simulink model "Cooperative"  (R2023b)
settings: Solver=FixedStepAuto  StartTime=0.0  StopTime=Sim_time  FixedStep=dt  RelTol=1e-3
values from neighbouring files (symbols this model uses):
  delta_r_max = 30*pi/180    (= 0.523598775598)    [Run_Cooperation.m]
  DS = 1    [Run_Cooperation.m]
  M_psi_r = 20*pi/180    (= 0.349065850399)    [Run_Cooperation.m]
  MaxF = 45    [Run_Cooperation.m]
  MinF = 15    [Run_Cooperation.m]
  SR = 30    [Run_Cooperation.m]
  targetX = [100,110,80,95]    [Run_Cooperation.m]
  targetY = [100, 120,130,125]    [Run_Cooperation.m]
  tau_s = 1    [Run_Cooperation.m]
  u0 = 1    [Run_Cooperation.m]
  xAUV_ini = [2, 15, 6, 20]    [Run_Cooperation.m]
  Xob = [35,50,80,50]    [Run_Cooperation.m]
  yAUV_ini = [15, -20, -5, 0]    [Run_Cooperation.m]
  Yob = [35,50,80,100]    [Run_Cooperation.m]
libraries: slpidlib x4, simulink x4
settings Model: Creator=Behnaz Hadi  LastModifiedBy=ps22aae
settings SolverCC: AlgebraicLoopSolver=TrustRegion
settings DataIOCC: ReturnWorkspaceOutputs=off
settings DebuggingCC: UnconnectedInputMsg=warning  UnconnectedOutputMsg=warning  UnconnectedLineMsg=warning  ArithmeticOperatorsInVariantConditions=warning
settings ModelReferenceCC: EnableRefExpFcnMdlSchedulingChecks=on
settings SFSimCC: CustomCodeUndefinedFunction=UseInterfaceOnly
settings RTWCC: DLArmComputeVersion=19.05

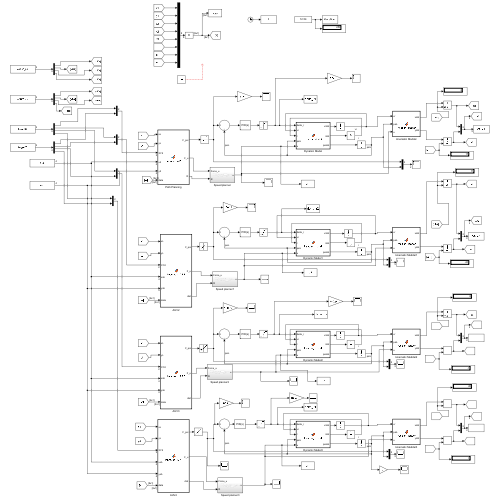
[thumbnail: Simulink's stored preview of the top-level diagram]
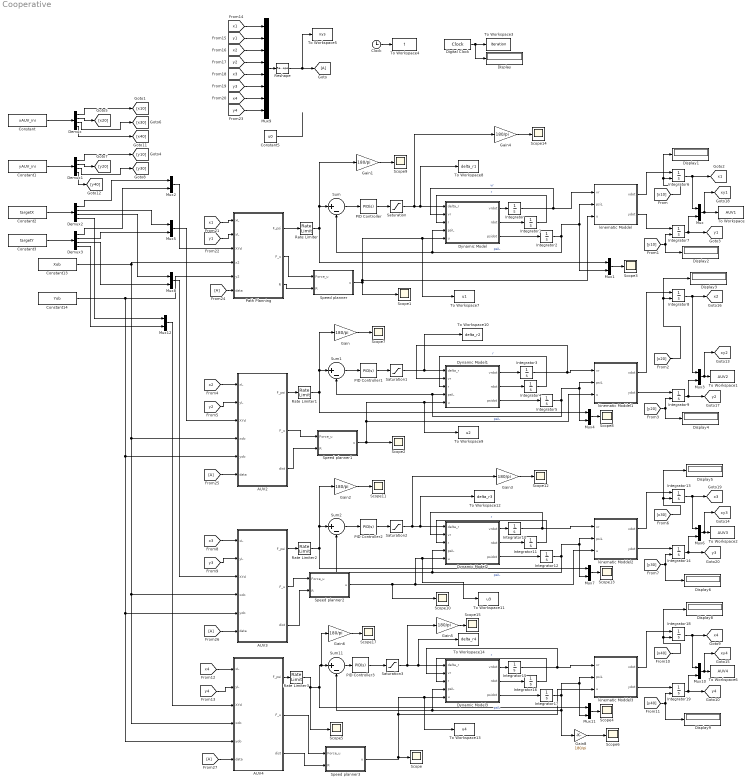
== system Cooperative ==
  AUV2 : MATLAB Function  TreatAsAtomicUnit=on
  AUV3 : MATLAB Function  TreatAsAtomicUnit=on
  AUV4 : MATLAB Function  TreatAsAtomicUnit=on
  Clock : Clock
  Constant : Constant  Value=xAUV_ini
  Constant1 : Constant  Value=yAUV_ini
  Constant13 : Constant  Value=Xob
  Constant14 : Constant  Value=Yob
  Constant2 : Constant  Value=targetX
  Constant3 : Constant  Value=targetY
  Constant5 : Constant  Value=u0
  Demux{,1..3} (4 alike) : Demux
  Digital Clock : DigitalClock
  Display{,1..6,8..9} (9 alike) : Display
  Dynamic Model : MATLAB Function  TreatAsAtomicUnit=on
  Dynamic Model1 : MATLAB Function  TreatAsAtomicUnit=on
  Dynamic Model2 : MATLAB Function  TreatAsAtomicUnit=on
  Dynamic Model3 : MATLAB Function  TreatAsAtomicUnit=on
  From{24..27} (4 alike) : From
  Gain{,1..6,8} (8 alike) : Gain  Gain=180/pi
  Goto : Goto
  Integrator{,1,3..4,10..11,15..16} (8 alike) : Integrator
  Integrator{2,5,12,17} (4 alike) : Integrator  InitialCondition=pi/6
  Integrator{6,8,13,18} (4 alike) : Integrator  InitialConditionSource=external  InitialCondition=6
  Integrator{7,9,14,19} (4 alike) : Integrator  InitialConditionSource=external  InitialCondition=4
  Mux{,1..8,10..12} (12 alike) : Mux  Inputs=2
  Mux9 : Mux  Inputs=8
  PID Controller{,1..3} (4 alike) : slpidlib/PID Controller  Controller=PID  Form=Ideal  TimeDomain=Continuous-time  UseExternalTs=off  SampleTime=-1  IntegratorMethod=Forward Euler  FilterMethod=Forward Euler  ControllerParametersSource=internal  P=-4.58375331776641  I=0.348826037798542  UseKiTs=off  D=0.667672634240164  N=10.0336095861132  UseFilter=on  TunerSelectOption=Transfer Function Based (PID Tuner App)  InitialConditionSource=internal  InitialConditionForIntegrator=0  InitialConditionForFilter=0  DifferentiatorICPrevScaledInput=0  ExternalReset=none  TrackingMode=off  Kt=1  LimitOutput=off  SatLimitsSource=internal  UpperSaturationLimit=inf  LowerSaturationLimit=-inf  LinearizeAsGain=on  AntiWindupMode=none  Kb=1  LimitIntegrator=off  UpperIntegratorSaturationLimit=inf  LowerIntegratorSaturationLimit=-inf  POutMin=[]  POutMax=[]  IOutMin=[]  IOutMax=[]  DOutMin=[]  DOutMax=[]  NOutMin=[]  NOutMax=[]  SumOutMin=[]  SumOutMax=[]  SaturationOutMin=[]  SaturationOutMax=[]  PParamMin=[]  PParamMax=[]  IParamMin=[]  IParamMax=[]  DParamMin=[]  DParamMax=[]  NParamMin=[]  NParamMax=[]  KbParamMin=[]  KbParamMax=[]  KtParamMin=[]  KtParamMax=[]  KbOutMin=[]  KbOutMax=[]  KtOutMin=[]  KtOutMax=[]  IntegratorOutMin=[]  IntegratorOutMax=[]  FilterOutMin=[]  FilterOutMax=[]  SumI1OutMin=[]  SumI1OutMax=[]  SumI2OutMin=[]  SumI2OutMax=[]  SumI3OutMin=[]  SumI3OutMax=[]  SumI4OutMin=[]  SumI4OutMax=[]  SumDOutMin=[]  SumDOutMax=[]  DifferentiatorOutMin=[]  DifferentiatorOutMax=[]  FilterDiffOutCoefMin=[]  FilterDiffOutCoefMax=[]  ReciprocalOutMin=[]  ReciprocalOutMax=[]  SumDenOutMin=[]  SumDenOutMax=[]  SumNumOutMin=[]  SumNumOutMax=[]  DivideOutMin=[]  DivideOutMax=[]  UdiffTsProdOutMin=[]  UdiffTsProdOutMax=[]  NTsProdOutMin=[]  NTsProdOutMax=[]  UintegralTsProdOutMin=[]  UintegralTsProdOutMax=[]  UngainTsProdOutMin=[]  UngainTsProdOutMax=[]  ClampingZeroOutDataTypeStr=Inherit: Inherit via back propagation  ClampingZeroOutMin=[]  ClampingZeroOutMax=[]  FilterDenConstantOutDataTypeStr=Inherit: Inherit via back propagation  FilterDenConstantOutMin=[]  FilterDenConstantOutMax=[]  PCopyOutDataTypeStr=Inherit: Inherit via back propagation  PCopyOutMin=[]  PCopyOutMax=[]  NCopyOutDataTypeStr=Inherit: Inherit via back propagation  NCopyOutMin=[]  NCopyOutMax=[]  IntegratorContinuousStateAttributes=''  IntegratorStateMustResolveToSignalObject=off  IntegratorRTWStateStorageClass=Auto  FilterContinuousStateAttributes=''  FilterStateMustResolveToSignalObject=off  FilterRTWStateStorageClass=Auto  ParallelPVariant=Passthrough  IdealPVariant=InternalParameters  IVariant=InternalParameters  DVariant=InternalParameters  IntegratorVariant=Continuous  SatVariant=Disabled  AWVariant=Passthrough  PCopyVariant=Disabled  TRVariant=Disabled  FdbkBlocksVariant=Forward  IdealPFdbkVariant=Disabled  SatFdbkVariant=Disabled  DerivativeFilterVariant=ContFilter  NVariant=InternalParameters  NCopyVariant=Disabled  FilterICVariant=InternalICsFilter  IntegratorICVariant=InternalICs  ExternalResetVariant=Disabled  TRSumVariant=Passthrough  SumFdbkVariant=Disabled  SumVariant=Sum_PID  TsampFilterVariant=InternalTs  TsampNgainVariant=Passthrough  TsampIntegralVariant=Disabled_SignalSpec  ExternalSaturationOutDataTypeStr=Inherit: Same as second input
  Path Planning : MATLAB Function  TreatAsAtomicUnit=on
  Rate Limiter{,1..3} (4 alike) : RateLimiter  RisingSlewLimit=M_psi_r  FallingSlewLimit=-M_psi_r  SampleTimeMode=inherited
  Reshape : Reshape  OutputDimensionality=Customize  OutputDimensions=[8,1]
  Saturation{,1..3} (4 alike) : Saturate  UpperLimit=delta_r_max  LowerLimit=-delta_r_max
  Scope{,1..15,17} (17 alike) : Scope
  Speed planner : Subsystem
  Speed planner1 : Subsystem
  Speed planner2 : Subsystem
  Speed planner3 : Subsystem
  Sum{,1..2,11} (4 alike) : Sum  Inputs=|+-
  To Workspace : ToWorkspace  VariableName=AUV1  SaveFormat=Structure With Time  SampleTime=-1
  To Workspace1 : ToWorkspace  VariableName=AUV2  SaveFormat=Structure With Time  SampleTime=-1
  To Workspace10 : ToWorkspace  VariableName=delta_r2  SampleTime=-1
  To Workspace11 : ToWorkspace  VariableName=u3  SampleTime=-1
  To Workspace12 : ToWorkspace  VariableName=delta_r3  SampleTime=-1
  To Workspace13 : ToWorkspace  VariableName=u4  SampleTime=-1
  To Workspace14 : ToWorkspace  VariableName=delta_r4  SampleTime=-1
  To Workspace2 : ToWorkspace  VariableName=AUV3  SaveFormat=Structure With Time  SampleTime=-1
  To Workspace3 : ToWorkspace  VariableName=iteration  SampleTime=-1
  To Workspace4 : ToWorkspace  VariableName=t  SampleTime=-1
  To Workspace5 : ToWorkspace  VariableName=xys  SampleTime=-1
  To Workspace6 : ToWorkspace  VariableName=AUV4  SaveFormat=Structure With Time  SampleTime=-1
  To Workspace7 : ToWorkspace  VariableName=u1  SampleTime=-1
  To Workspace8 : ToWorkspace  VariableName=delta_r1  SampleTime=-1
  To Workspace9 : ToWorkspace  VariableName=u2  SampleTime=-1
  kinematic Moddel : MATLAB Function  TreatAsAtomicUnit=on
  kinematic Moddel1 : MATLAB Function  TreatAsAtomicUnit=on
  kinematic Moddel2 : MATLAB Function  TreatAsAtomicUnit=on
  kinematic Moddel3 : MATLAB Function  TreatAsAtomicUnit=on
  tag scope: x1=global, x2=global, x3=global, x4=global, xy1=global, xy2=global, xy3=global, xy4=global, y1=global, y2=global, y3=global, y4=global
  wires:
  [x1] -> Path Planning/1(xL)
  [y1] -> Path Planning/2(yL)
  kinematic Moddel/1(xdot) -> Integrator6/1
  Integrator6/1 -> [x1], Mux/1
  kinematic Moddel/2(ydot) -> Integrator7/1
  Mux1/1 -> Scope3/1
  Integrator1/1 -> Dynamic Model/3(r)  "r"
  Dynamic Model/1(vrdot) -> Integrator/1
  PID Controller/1 -> Saturation/1
  Dynamic Model/3(psidot) -> Integrator2/1
  Integrator2/1 -> Mux1/2, kinematic Moddel/2(psiL), Dynamic Model/4(psiL), Sum/2  "psiL"
  Sum/1 -> PID Controller/1
  Integrator/1 -> Dynamic Model/2(vr), kinematic Moddel/1(vr)  "vr"
  Mux/1 -> [xy1], To Workspace/1
  Dynamic Model/2(rdot) -> Integrator1/1
  Clock/1 -> To Workspace4/1
  Digital Clock/1 -> Display/1, To Workspace3/1
  Path Planning/1(F_psi) -> Rate Limiter/1
  Constant/1 -> Demux/1
  Constant1/1 -> Demux1/1
  Demux/1 -> [x10]
  [x10] -> Display1/1, Integrator6/2
  [y10] -> Integrator7/2, Display2/1
  Demux/2 -> [x20]
  Demux/3 -> [x30]
  Demux1/2 -> [y20]
  Demux1/1 -> [y10]
  Demux1/3 -> [y30]
  Demux2/2 -> Mux5/1
  Demux2/1 -> Mux2/1
  Demux2/3 -> Mux8/1
  Demux3/3 -> Mux8/2
  Demux3/1 -> Mux2/2
  Mux2/1 -> Path Planning/3(XYd)
  [y20] -> Integrator9/2, Display4/1
  AUV2/1(F_psi) -> Rate Limiter1/1
  Sum1/1 -> PID Controller1/1
  Mux3/1 -> [xy2], To Workspace1/1
  Dynamic Model1/2(rdot) -> Integrator4/1
  Dynamic Model1/3(psidot) -> Integrator5/1
  Mux4/1 -> Scope8/1
  Integrator8/1 -> Mux3/1, [x2]
  [y2] -> AUV2/2(yL)
  Integrator4/1 -> Dynamic Model1/3(r)  "r"
  kinematic Moddel1/2(ydot) -> Integrator9/1
  Integrator9/1 -> Mux3/2, [y2]
  kinematic Moddel1/1(xdot) -> Integrator8/1
  Mux5/1 -> AUV2/3(XYd)
  [x20] -> Display3/1, Integrator8/2
  Integrator5/1 -> Mux4/2, kinematic Moddel1/2(psiL), Dynamic Model1/4(psiL), Sum1/2  "psiL"
  PID Controller1/1 -> Saturation1/1
  [x2] -> AUV2/1(xL)
  Dynamic Model1/1(vrdot) -> Integrator3/1
  Integrator11/1 -> Dynamic Model2/3(r)  "r"
  Sum2/1 -> PID Controller2/1
  [y30] -> Integrator14/2, Display6/1
  AUV3/1(F_psi) -> Rate Limiter2/1
  Mux6/1 -> [xy3], To Workspace2/1
  [y3] -> AUV3/2(yL)
  [x3] -> AUV3/1(xL)
  Dynamic Model2/2(rdot) -> Integrator11/1
  Integrator12/1 -> Mux7/2, kinematic Moddel2/2(psiL), Dynamic Model2/4(psiL), Sum2/2  "psiL"
  Dynamic Model2/3(psidot) -> Integrator12/1
  kinematic Moddel2/2(ydot) -> Integrator14/1
  Integrator14/1 -> Mux6/2, [y3]
  PID Controller2/1 -> Saturation2/1
  Integrator13/1 -> Mux6/1, [x3]
  Mux7/1 -> Scope13/1
  [x30] -> Display5/1, Integrator13/2
  kinematic Moddel2/1(xdot) -> Integrator13/1
  Dynamic Model2/1(vrdot) -> Integrator10/1
  Demux3/2 -> Mux5/2
  Speed planner1/1(u) -> To Workspace9/1, Dynamic Model1/5(u), kinematic Moddel1/3(u), Scope2/1
  AUV3/3(dist) -> Speed planner2/2(R)
  Speed planner2/1(u) -> kinematic Moddel2/3(u), To Workspace11/1, Dynamic Model2/5(u), Scope10/1
  Integrator7/1 -> [y1], Mux/2
  Constant2/1 -> Demux2/1
  Constant3/1 -> Demux3/1
  Sum11/1 -> PID Controller3/1
  Integrator16/1 -> Dynamic Model3/3(r)  "r"
  Mux11/1 -> Scope4/1
  Integrator18/1 -> Mux10/1, [x4]
  Dynamic Model3/1(vrdot) -> Integrator15/1
  kinematic Moddel3/1(xdot) -> Integrator18/1
  [x40] -> Display8/1, Integrator18/2
  Integrator19/1 -> Mux10/2, [y4]
  Integrator17/1 -> Gain8/1, Dynamic Model3/4(psiL), Sum11/2, Mux11/2, kinematic Moddel3/2(psiL)  "psiL"
  kinematic Moddel3/2(ydot) -> Integrator19/1
  PID Controller3/1 -> Saturation3/1
  Dynamic Model3/3(psidot) -> Integrator17/1
  Dynamic Model3/2(rdot) -> Integrator16/1
  [y4] -> AUV4/2(yL)
  [x4] -> AUV4/1(xL)
  Mux10/1 -> [xy4], To Workspace6/1
  AUV4/3(dist) -> Speed planner3/2(R)
  [y40] -> Integrator19/2, Display9/1
  Demux/4 -> [x40]
  Demux1/4 -> [y40]
  Demux2/4 -> Mux12/1
  Demux3/4 -> Mux12/2
  Mux12/1 -> AUV4/3(XYd)
  Constant13/1 -> AUV4/4(xob), AUV3/4(xob), AUV2/4(xob), Path Planning/4(x2)
  Constant14/1 -> AUV4/5(yob), AUV3/5(yob), AUV2/5(yob), Path Planning/5(y2)
  Mux8/1 -> AUV3/3(XYd)
  [x1] -> Mux9/1
  [y1] -> Mux9/2
  [y2] -> Mux9/4
  [x2] -> Mux9/3
  [y3] -> Mux9/6
  [x3] -> Mux9/5
  [y4] -> Mux9/8
  [x4] -> Mux9/7
  From24/1 -> Path Planning/6(data)
  Mux9/1 -> Reshape/1
  Reshape/1 -> To Workspace5/1, Goto/1
  From25/1 -> AUV2/6(data)
  From26/1 -> AUV3/6(data)
  From27/1 -> AUV4/6(data)
  Gain8/1 -> Scope6/1
  Constant5/1 -> ?
  Integrator3/1 -> Dynamic Model1/2(vr), kinematic Moddel1/1(vr)
  Speed planner/1(u) -> Scope1/1, To Workspace7/1, Dynamic Model/5(u), kinematic Moddel/3(u)
  Path Planning/2(F_u) -> Speed planner/1(Force_u)
  Path Planning/3(R) -> Speed planner/2(R)
  AUV2/3(dist) -> Speed planner1/2(R)
  AUV2/2(F_u) -> Speed planner1/1(Force_u)
  Gain/1 -> Scope7/1
  Gain1/1 -> Scope9/1
  Rate Limiter/1 -> Mux1/1, Gain1/1, Sum/1
  Rate Limiter1/1 -> Mux4/1, Gain/1, Sum1/1
  Integrator10/1 -> Dynamic Model2/2(vr), kinematic Moddel2/1(vr)
  AUV3/2(F_u) -> Speed planner2/1(Force_u)
  Gain2/1 -> Scope11/1
  Rate Limiter2/1 -> Mux7/1, Gain2/1, Sum2/1
  Gain3/1 -> Scope12/1
  Gain4/1 -> Scope14/1
  Saturation/1 -> Gain4/1, To Workspace8/1, Dynamic Model/1(delta_r)
  Saturation1/1 -> To Workspace10/1, Dynamic Model1/1(delta_r)
  Saturation2/1 -> Gain3/1, To Workspace12/1, Dynamic Model2/1(delta_r)
  Integrator15/1 -> Dynamic Model3/2(vr), kinematic Moddel3/1(vr)
  AUV4/2(F_u) -> Speed planner3/1(Force_u)
  Speed planner3/1(u) -> Scope/1, kinematic Moddel3/3(u), To Workspace13/1, Dynamic Model3/5(u)
  Gain5/1 -> Scope15/1
  Saturation3/1 -> Gain5/1, To Workspace14/1, Dynamic Model3/1(delta_r)
  Gain6/1 -> Scope17/1
  AUV4/1(F_psi) -> Rate Limiter3/1
  Rate Limiter3/1 -> Scope5/1, Gain6/1, Sum11/1, Mux11/1

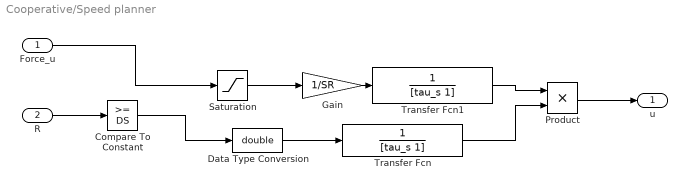
== system Cooperative/Speed planner ==
  Force_u : Inport
  R : Inport  Port=2
  Compare To Constant : simulink/Logic and Bit Operations/Compare To Constant  relop=>=  const=DS  OutDataTypeStr=boolean
  Data Type Conversion : DataTypeConversion  OutDataTypeStr=double  SaturateOnIntegerOverflow=off  RndMeth=Floor
  Gain : Gain  Gain=1/SR
  Product : Product
  Saturation : Saturate  UpperLimit=MaxF  LowerLimit=MinF
  Transfer Fcn : TransferFcn  Denominator=[tau_s 1]
  Transfer Fcn1 : TransferFcn  Denominator=[tau_s 1]
  u : Outport
  wires:
  Compare To Constant/1 -> Data Type Conversion/1
  Saturation/1 -> Gain/1
  Product/1 -> u/1
  Gain/1 -> Transfer Fcn1/1
  Transfer Fcn/1 -> Product/2
  Transfer Fcn1/1 -> Product/1
  R/1 -> Compare To Constant/1
  Data Type Conversion/1 -> Transfer Fcn/1
  Force_u/1 -> Saturation/1

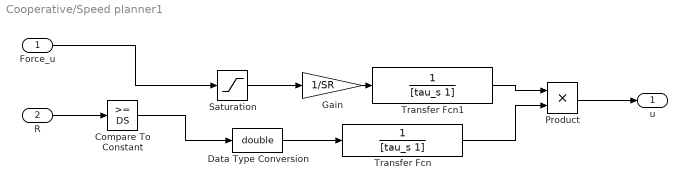
== system Cooperative/Speed planner1 ==
  Force_u : Inport
  R : Inport  Port=2
  Compare To Constant : simulink/Logic and Bit Operations/Compare To Constant  relop=>=  const=DS  OutDataTypeStr=boolean
  Data Type Conversion : DataTypeConversion  OutDataTypeStr=double  SaturateOnIntegerOverflow=off  RndMeth=Floor
  Gain : Gain  Gain=1/SR
  Product : Product
  Saturation : Saturate  UpperLimit=MaxF  LowerLimit=MinF
  Transfer Fcn : TransferFcn  Denominator=[tau_s 1]
  Transfer Fcn1 : TransferFcn  Denominator=[tau_s 1]
  u : Outport
  wires:
  Compare To Constant/1 -> Data Type Conversion/1
  Saturation/1 -> Gain/1
  Product/1 -> u/1
  Gain/1 -> Transfer Fcn1/1
  Transfer Fcn/1 -> Product/2
  Transfer Fcn1/1 -> Product/1
  R/1 -> Compare To Constant/1
  Data Type Conversion/1 -> Transfer Fcn/1
  Force_u/1 -> Saturation/1

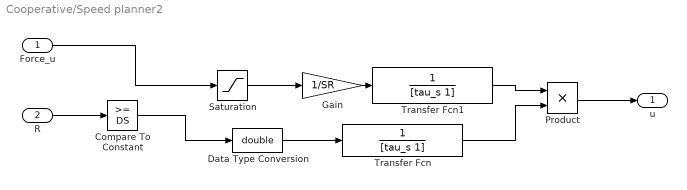
== system Cooperative/Speed planner2 ==
  Force_u : Inport
  R : Inport  Port=2
  Compare To Constant : simulink/Logic and Bit Operations/Compare To Constant  relop=>=  const=DS  OutDataTypeStr=boolean
  Data Type Conversion : DataTypeConversion  OutDataTypeStr=double  SaturateOnIntegerOverflow=off  RndMeth=Floor
  Gain : Gain  Gain=1/SR
  Product : Product
  Saturation : Saturate  UpperLimit=MaxF  LowerLimit=MinF
  Transfer Fcn : TransferFcn  Denominator=[tau_s 1]
  Transfer Fcn1 : TransferFcn  Denominator=[tau_s 1]
  u : Outport
  wires:
  Compare To Constant/1 -> Data Type Conversion/1
  Saturation/1 -> Gain/1
  Product/1 -> u/1
  Gain/1 -> Transfer Fcn1/1
  Transfer Fcn/1 -> Product/2
  Transfer Fcn1/1 -> Product/1
  R/1 -> Compare To Constant/1
  Data Type Conversion/1 -> Transfer Fcn/1
  Force_u/1 -> Saturation/1

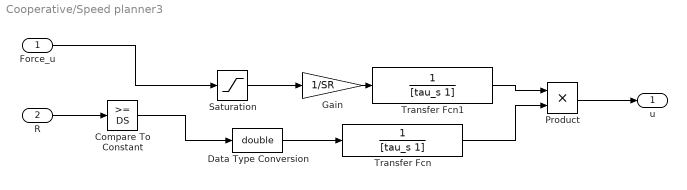
== system Cooperative/Speed planner3 ==
  Force_u : Inport
  R : Inport  Port=2
  Compare To Constant : simulink/Logic and Bit Operations/Compare To Constant  relop=>=  const=DS  OutDataTypeStr=boolean
  Data Type Conversion : DataTypeConversion  OutDataTypeStr=double  SaturateOnIntegerOverflow=off  RndMeth=Floor
  Gain : Gain  Gain=1/SR
  Product : Product
  Saturation : Saturate  UpperLimit=MaxF  LowerLimit=MinF
  Transfer Fcn : TransferFcn  Denominator=[tau_s 1]
  Transfer Fcn1 : TransferFcn  Denominator=[tau_s 1]
  u : Outport
  wires:
  Compare To Constant/1 -> Data Type Conversion/1
  Saturation/1 -> Gain/1
  Product/1 -> u/1
  Gain/1 -> Transfer Fcn1/1
  Transfer Fcn/1 -> Product/2
  Transfer Fcn1/1 -> Product/1
  R/1 -> Compare To Constant/1
  Data Type Conversion/1 -> Transfer Fcn/1
  Force_u/1 -> Saturation/1

== matlab function Cooperative/Dynamic Model2 ==
  data: delta_r input; vrdot output; vr input; r input; psiL input; rdot output; psidot output; u input
function [vrdot,rdot,psidot] = Leader_Model(delta_r,vr,r,psiL,u)
% global U0
U0 = u;
m = 30.48;        %kg
Y_vrdot = -35.5;  %kg
Y_rdot = 1.93;    %kg/rad
Y_vr = -66.6;
Y_r = 2.2;        % kgm/s
N_vrdot = 1.93;   % kgm
N_rdot = -4.88;   % kgm2/rad
N_vr = -4.47;     % kgm/s
N_r = -6.87;      % kgm2/s
N_delta = -34.6/3.5;
Y_delta = 50.6/3.5;
Izz = 3.45;       % kgm2/rad 
x_state = [vr;r;psiL];
% xdot_state = inv([m-Y_vrdot -Y_rdot 0; -N_vrdot Izz-N_rdot 0; 0 0 1])*...
%                  [Y_vr Y_r-m*U0 0;N_vr N_r 0; 0 1 0]*x_state+...
%              inv([m-Y_vrdot -Y_rdot 0; -N_vrdot Izz-N_rdot 0; 0 0 1])*[Y_delta;N_delta;0]*delta_r;
A =inv([m-Y_vrdot -Y_rdot  0;...
       -N_vrdot Izz-N_rdot 0; ...
        0          0       1]);
B=[Y_vr Y_r-m*U0 0;...
   N_vr   N_r    0;...
    0     1      0];
C=A*B;
D=A*[Y_delta;N_delta;0];

states_vector = A*B*x_state + A*[Y_delta;N_delta;0]*delta_r;
  
vrdot = states_vector(1); rdot = states_vector(2);
psidot = states_vector(3);
%     vrdot  = C(1,1)*x_state(1)+ C(1,2)*x_state(2)+D(1)*delta_r ;  %vr_dot
%     rdot  =  C(2,1)*x_state(1)+ C(2,2)*x_state(2)+D(2)*delta_r ;  %r_dot
%     sadot  = x_state(2) ;  %sa_dot
%     xx(4) = xx(3)*180/pi;
%     
% 
%     if xx(3)> pi
%         xx(3)= xx(3)-2*pi;
%     end
%     if xx(3) < -pi
%         xx(3)= xx(3)+2*pi;
%     end    
end

== matlab function Cooperative/AUV4 ==
  data: xL input; F_psi output; F_u output; yL input; XYd input; dist output; xob input; yob input; data input
function [F_psi, F_u, dist] = improved_APF(xL, yL, XYd, xob, yob, data)
% Improved APF for multiple AUVs, handling forces from 4 obstacles

% Constants
p0 = 10; kp = 1; m = 80; R = 5; N = 2;
numAUVs = length(xL); % Number of AUVs (4)

% Goal and robot positions
Xd = [XYd(1); XYd(2)];  % Goal position (same for all AUVs)
XL = [xL; yL];  % Leader positions (one for each AUV)

Rat = norm(Xd - XL);  % Distance to goal

% Initialize output arrays for AUVs
F_psi = zeros(numAUVs, 1);
F_u = zeros(numAUVs, 1);
dist = zeros(numAUVs, 1);

% First repulsion layer (obstacles)
Xobs = [xob(:)'; yob(:)'];
Frep = zeros(2, 4);  % Repulsion force matrix for 4 obstacles

for i = 1:numAUVs
    % For each AUV, calculate the distance to obstacles and apply repulsion
    for j = 1:4
        obs = Xobs(:,j);
        Rrep = norm(obs - XL(:,i)) - R;
        if Rrep <= p0
            F1 = ((1/Rrep) - (1/p0)) * (-(Rat^N)/(Rrep^2));
            F2 = ((1/Rrep) - (1/p0))^2 * (Rat^(N-1));
            Fmag = m*F1 + (N/2)*m*F2;
            dir = atan2(obs(2)-XL(2,i), obs(1)-XL(1,i));
            Frep(:,j) = Fmag * [cos(dir); sin(dir)];
        end
    end
    
    % Calculate total repulsion force for AUV i
    Frep_total = sum(Frep, 2);

    % Calculate attraction force (same goal for all AUVs)
    Fatt = kp * Rat;
    alfa = atan2(Xd(2)-XL(2,i), Xd(1)-XL(1,i));
    Fatt_vec = Fatt * [cos(alfa); sin(alfa)];

    % Total force
    F_total = Frep_total + Fatt_vec;
    F_psi(i) = atan2(F_total(2), F_total(1));  % Heading for AUV i
    F_u(i) = norm(F_total);  % Speed magnitude for AUV i
    dist(i) = norm(Xd - XL(:,i));  % Distance to goal for AUV i
end

end

== matlab function Cooperative/Path Planning ==
  data: xL input; F_psi output; F_u output; yL input; XYd input; R output; x2 input; y2 input; data input
%%%%%%%%%%%% Classic APF Sample, uncomment if needed %%%%%%%%%%%%%%%%%%%%%%
%%%%%%%%%%%%%%%%%%%%%%%%%%%%%%%%%%%%%%%%%%%%%%%%%%%%%%%%%%%%%%%%%%%%%%%%%%%
% function [F_psi, F_u, R] = improved_APF(xL, yL, XYd, x2, y2, data)
%     % Parameters
%     K_att = 1.0;              % Attractive gain (same)
%     K_rep_static = 100;       % Repulsive gain for static obstacles
%     K_rep_dyn = 100;          % Stronger repulsion for dynamic (moving) AUVs
%     rho_0_static = 15;        % Influence range for static
%     rho_0_dyn = 15;           % Influence range for dynamic
%     R_static = 8;             % Obstacle radius for static
%     R_dyn = 4;                % Obstacle radius for dynamic
% 
%     % Positions
%     XL = [xL; yL];            % Agent position
%     Xd = [XYd(1); XYd(2)];    % Goal position
%     Xobs = [x2(:)'; y2(:)'];  % Static obstacles (AUVs)
%     R = norm(Xd - XL);        % Distance to goal
% 
%     % Attractive force
%     Fatt = -K_att * (XL - Xd);
% 
%     % Repulsive force: static (4 agents)
%     Frep_total = [0; 0];
%     for i = 1:4
%         obs = Xobs(:, i);
%         rho = norm(XL - obs) - R_static;
%         if rho <= rho_0_static
%             diff = XL - obs;
%             Frep = K_rep_static * (1/rho - 1/rho_0_static) * (diff / rho^3);
%             Frep_total = Frep_total + Frep;
%         end
%     end
% 
%     % Repulsive force: dynamic obstacles from data
%     for i = 1:3
%         obs = data((2*i+1):(2*i+2));
%         rho = norm(XL - obs) - R_dyn;
%         if rho <= rho_0_dyn
%             diff = XL - obs;
%             Frep = K_rep_dyn * (1/rho - 1/rho_0_dyn) * (diff / rho^3);
%             Frep_total = Frep_total + Frep;
%         end
%     end
% 
%     % Total force and outputs
%     F_total = Fatt + Frep_total;
%     F_psi = atan2(F_total(2), F_total(1));
%     F_u = norm(F_total);
% end

function [F_psi, F_u, R] = improved_APF(xL, yL, XYd, x2, y2, data)
    %% APF Parameters
    % First layer repulsion
    p0 = 15; kp = 1; m = 70; R0 = 5; N = 2;

    % Goal and agent position
    Xd = [XYd(1); XYd(2)];     % Desired goal
    XL = [xL; yL];             % Agent position

    % Obstacles (other AUVs)
    Xobs = [x2(:)'; y2(:)'];   % Each column is [x; y] of an obstacle
    Rat = norm(Xd - XL);       % Distance to goal

    %% Compute repulsion from each obstacle (first layer)
    Frep_total = [0; 0];
    for i = 1:4
        obs = Xobs(:, i);
        Rrep = norm(obs - XL) - R0;

        if Rrep <= p0
            F1 = ((1/Rrep) - (1/p0)) * (-(Rat^N) / (Rrep^2));
            F2 = ((1/Rrep - 1/p0)^2) * (Rat^(N - 1));
            Frep_mag = m * F1 + (N/2) * m * F2;

            dir = obs - XL;
            beta = atan2(dir(2), dir(1));
            Frep = Frep_mag * [cos(beta); sin(beta)];

            Frep_total = Frep_total + Frep;
        end
    end

    %% Second layer repulsion (from `data`)
    % Updated parameters
    p0 = 10; kp = 1.5; m = 5; R0 = 2;

    for i = 1:3
        obs = data((2*i+1):(2*i+2));
        Rrep = norm(obs - XL) - R0;

        if Rrep <= p0
            F1 = ((1/Rrep) - (1/p0)) * (-(Rat^N) / (Rrep^2));
            F2 = ((1/Rrep - 1/p0)^2) * (Rat^(N - 1));
            Frep_mag = m * F1 + (N/2) * m * F2;

            dir = obs - XL;
            beta = atan2(dir(2), dir(1));
            Frep = Frep_mag * [cos(beta); sin(beta)];

            Frep_total = Frep_total + Frep;
        end
    end

    %% Compute attractive force
    Fatt_mag = kp * Rat;
    direction_to_goal = Xd - XL;
    alpha = atan2(direction_to_goal(2), direction_to_goal(1));
    Fatt = Fatt_mag * [cos(alpha); sin(alpha)];

    %% Resulting force vector
    F_total = Frep_total + Fatt;

    %% Output
    F_psi = atan2(F_total(2), F_total(1));      % Direction of total force
    F_u = norm(F_total);                        % Magnitude of total force
    R = Rat;                                    % Distance to goal
end

== matlab function Cooperative/kinematic Moddel2 ==
  data: vr input; psiL input; xdot output; ydot output; u input
function [xdot,ydot] = Position_leader(vr,psiL,u)
% global U0
U0 = u;
% Ucx =0.2; Ucy =0.2; 
Ucx =0.0; Ucy =0.0; 
% Ucx =0.2; Ucy =0.2; 


% x_dot = U0*cos(sa) - vr*sin(sa)+Ucx;
% y_dot = U0*sin(sa) + vr*cos(sa)+Ucy;
xdot  = U0*cos(psiL) - vr*sin(psiL)+ Ucx ;  %x_dot
ydot  = U0*sin(psiL) + vr*cos(psiL)+ Ucy ;  %y_dot

end

== matlab function Cooperative/Dynamic Model3 ==
  data: delta_r input; vrdot output; vr input; r input; psiL input; rdot output; psidot output; u input
function [vrdot,rdot,psidot] = Leader_Model(delta_r,vr,r,psiL,u)
% global U0
U0 = u;
m = 30.48;        %kg
Y_vrdot = -35.5;  %kg
Y_rdot = 1.93;    %kg/rad
Y_vr = -66.6;
Y_r = 2.2;        % kgm/s
N_vrdot = 1.93;   % kgm
N_rdot = -4.88;   % kgm2/rad
N_vr = -4.47;     % kgm/s
N_r = -6.87;      % kgm2/s
N_delta = -34.6/3.5;
Y_delta = 50.6/3.5;
Izz = 3.45;       % kgm2/rad 
x_state = [vr;r;psiL];
% xdot_state = inv([m-Y_vrdot -Y_rdot 0; -N_vrdot Izz-N_rdot 0; 0 0 1])*...
%                  [Y_vr Y_r-m*U0 0;N_vr N_r 0; 0 1 0]*x_state+...
%              inv([m-Y_vrdot -Y_rdot 0; -N_vrdot Izz-N_rdot 0; 0 0 1])*[Y_delta;N_delta;0]*delta_r;
A =inv([m-Y_vrdot -Y_rdot  0;...
       -N_vrdot Izz-N_rdot 0; ...
        0          0       1]);
B=[Y_vr Y_r-m*U0 0;...
   N_vr   N_r    0;...
    0     1      0];
C=A*B;
D=A*[Y_delta;N_delta;0];

states_vector = A*B*x_state + A*[Y_delta;N_delta;0]*delta_r;
  
vrdot = states_vector(1); rdot = states_vector(2);
psidot = states_vector(3);
%     vrdot  = C(1,1)*x_state(1)+ C(1,2)*x_state(2)+D(1)*delta_r ;  %vr_dot
%     rdot  =  C(2,1)*x_state(1)+ C(2,2)*x_state(2)+D(2)*delta_r ;  %r_dot
%     sadot  = x_state(2) ;  %sa_dot
%     xx(4) = xx(3)*180/pi;
%     
% 
%     if xx(3)> pi
%         xx(3)= xx(3)-2*pi;
%     end
%     if xx(3) < -pi
%         xx(3)= xx(3)+2*pi;
%     end    
end

== matlab function Cooperative/kinematic Moddel3 ==
  data: vr input; psiL input; xdot output; ydot output; u input
function [xdot,ydot] = Position_leader(vr,psiL,u)
% global U0
U0 = u;
% Ucx =0.2; Ucy =0.2; 
Ucx =0.0; Ucy =0.0; 
% Ucx =0.2; Ucy =0.2; 


% x_dot = U0*cos(sa) - vr*sin(sa)+Ucx;
% y_dot = U0*sin(sa) + vr*cos(sa)+Ucy;
xdot  = U0*cos(psiL) - vr*sin(psiL)+ Ucx ;  %x_dot
ydot  = U0*sin(psiL) + vr*cos(psiL)+ Ucy ;  %y_dot

end

== matlab function Cooperative/kinematic Moddel ==
  data: vr input; psiL input; xdot output; ydot output; u input
function [xdot,ydot] = Position_leader(vr,psiL,u)
% global U0
U0 = u;
% Ucx =0.2; Ucy =0.2; 
Ucx =0.0; Ucy =0.0; 
% Ucx =0.2; Ucy =0.2; 


% x_dot = U0*cos(sa) - vr*sin(sa)+Ucx;
% y_dot = U0*sin(sa) + vr*cos(sa)+Ucy;
xdot  = U0*cos(psiL) - vr*sin(psiL)+ Ucx ;  %x_dot
ydot  = U0*sin(psiL) + vr*cos(psiL)+ Ucy ;  %y_dot

end

== matlab function Cooperative/Dynamic Model ==
  data: delta_r input; vrdot output; vr input; r input; psiL input; rdot output; psidot output; u input
function [vrdot,rdot,psidot] = Leader_Model(delta_r,vr,r,psiL,u)
% global U0
U0 =u;
m = 30.48;        %kg
Y_vrdot = -35.5;  %kg
Y_rdot = 1.93;    %kg/rad
Y_vr = -66.6;
Y_r = 2.2;        % kgm/s
N_vrdot = 1.93;   % kgm
N_rdot = -4.88;   % kgm2/rad
N_vr = -4.47;     % kgm/s
N_r = -6.87;      % kgm2/s
N_delta = -34.6/3.5;
Y_delta = 50.6/3.5;
Izz = 3.45;       % kgm2/rad 
x_state = [vr;r;psiL];
% xdot_state = inv([m-Y_vrdot -Y_rdot 0; -N_vrdot Izz-N_rdot 0; 0 0 1])*...
%                  [Y_vr Y_r-m*U0 0;N_vr N_r 0; 0 1 0]*x_state+...
%              inv([m-Y_vrdot -Y_rdot 0; -N_vrdot Izz-N_rdot 0; 0 0 1])*[Y_delta;N_delta;0]*delta_r;
A =inv([m-Y_vrdot -Y_rdot  0;...
       -N_vrdot Izz-N_rdot 0; ...
        0          0       1]);
B=[Y_vr Y_r-m*U0 0;...
   N_vr   N_r    0;...
    0     1      0];
C=A*B;
D=A*[Y_delta;N_delta;0];

states_vector = A*B*x_state + A*[Y_delta;N_delta;0]*delta_r;
  
vrdot = states_vector(1); rdot = states_vector(2);
psidot = states_vector(3);
%     vrdot  = C(1,1)*x_state(1)+ C(1,2)*x_state(2)+D(1)*delta_r ;  %vr_dot
%     rdot  =  C(2,1)*x_state(1)+ C(2,2)*x_state(2)+D(2)*delta_r ;  %r_dot
%     sadot  = x_state(2) ;  %sa_dot
%     xx(4) = xx(3)*180/pi;
%     
% 
%     if xx(3)> pi
%         xx(3)= xx(3)-2*pi;
%     end
%     if xx(3) < -pi
%         xx(3)= xx(3)+2*pi;
%     end    
end

== matlab function Cooperative/AUV2 ==
  data: xL input; F_psi output; F_u output; yL input; XYd input; dist output; xob input; yob input; data input
function [F_psi, F_u, dist] = improved_APF(xL, yL, XYd, xob, yob, data)
% Improved APF for multiple AUVs, handling forces from 4 obstacles

% Constants
p0 = 15; kp = 1; m = 90; R = 3; N = 2;
numAUVs = length(xL); % Number of AUVs (4)

% Goal and robot positions
Xd = [XYd(1); XYd(2)];  % Goal position (same for all AUVs)
XL = [xL; yL];  % Leader positions (one for each AUV)

Rat = norm(Xd - XL);  % Distance to goal

% Initialize output arrays for AUVs
F_psi = zeros(numAUVs, 1);
F_u = zeros(numAUVs, 1);
dist = zeros(numAUVs, 1);

% First repulsion layer (obstacles)
Xobs = [xob(:)'; yob(:)'];
Frep = zeros(2, 4);  % Repulsion force matrix for 4 obstacles

for i = 1:numAUVs
    % For each AUV, calculate the distance to obstacles and apply repulsion
    for j = 1:4
        obs = Xobs(:,j);
        Rrep = norm(obs - XL(:,i)) - R;
        if Rrep <= p0
            F1 = ((1/Rrep) - (1/p0)) * (-(Rat^N)/(Rrep^2));
            F2 = ((1/Rrep) - (1/p0))^2 * (Rat^(N-1));
            Fmag = m*F1 + (N/2)*m*F2;
            dir = atan2(obs(2)-XL(2,i), obs(1)-XL(1,i));
            Frep(:,j) = Fmag * [cos(dir); sin(dir)];
        end
    end
    
    % Calculate total repulsion force for AUV i
    Frep_total = sum(Frep, 2);

    % Calculate attraction force (same goal for all AUVs)
    Fatt = kp * Rat;
    alfa = atan2(Xd(2)-XL(2,i), Xd(1)-XL(1,i));
    Fatt_vec = Fatt * [cos(alfa); sin(alfa)];

    % Total force
    F_total = Frep_total + Fatt_vec;
    F_psi(i) = atan2(F_total(2), F_total(1));  % Heading for AUV i
    F_u(i) = norm(F_total);  % Speed magnitude for AUV i
    dist(i) = norm(Xd - XL(:,i));  % Distance to goal for AUV i
end

end

== matlab function Cooperative/Dynamic Model1 ==
  data: delta_r input; vrdot output; vr input; r input; psiL input; rdot output; psidot output; u input
function [vrdot,rdot,psidot] = Leader_Model(delta_r,vr,r,psiL,u)
% global U0
U0 =u;
m = 30.48;        %kg
Y_vrdot = -35.5;  %kg
Y_rdot = 1.93;    %kg/rad
Y_vr = -66.6;
Y_r = 2.2;        % kgm/s
N_vrdot = 1.93;   % kgm
N_rdot = -4.88;   % kgm2/rad
N_vr = -4.47;     % kgm/s
N_r = -6.87;      % kgm2/s
N_delta = -34.6/3.5;
Y_delta = 50.6/3.5;
Izz = 3.45;       % kgm2/rad 
x_state = [vr;r;psiL];
% xdot_state = inv([m-Y_vrdot -Y_rdot 0; -N_vrdot Izz-N_rdot 0; 0 0 1])*...
%                  [Y_vr Y_r-m*U0 0;N_vr N_r 0; 0 1 0]*x_state+...
%              inv([m-Y_vrdot -Y_rdot 0; -N_vrdot Izz-N_rdot 0; 0 0 1])*[Y_delta;N_delta;0]*delta_r;
A =inv([m-Y_vrdot -Y_rdot  0;...
       -N_vrdot Izz-N_rdot 0; ...
        0          0       1]);
B=[Y_vr Y_r-m*U0 0;...
   N_vr   N_r    0;...
    0     1      0];
C=A*B;
D=A*[Y_delta;N_delta;0];

states_vector = A*B*x_state + A*[Y_delta;N_delta;0]*delta_r;
  
vrdot = states_vector(1); rdot = states_vector(2);
psidot = states_vector(3);
%     vrdot  = C(1,1)*x_state(1)+ C(1,2)*x_state(2)+D(1)*delta_r ;  %vr_dot
%     rdot  =  C(2,1)*x_state(1)+ C(2,2)*x_state(2)+D(2)*delta_r ;  %r_dot
%     sadot  = x_state(2) ;  %sa_dot
%     xx(4) = xx(3)*180/pi;
%     
% 
%     if xx(3)> pi
%         xx(3)= xx(3)-2*pi;
%     end
%     if xx(3) < -pi
%         xx(3)= xx(3)+2*pi;
%     end    
end

== matlab function Cooperative/AUV3 ==
  data: xL input; F_psi output; F_u output; yL input; XYd input; dist output; xob input; yob input; data input
function [F_psi, F_u, dist] = improved_APF(xL, yL, XYd, xob, yob, data)
% Improved APF for multiple AUVs, handling forces from 4 obstacles

% Constants
p0 = 15; kp = 1; m = 70; R = 5; N = 2;
numAUVs = length(xL); % Number of AUVs (4)

% Goal and robot positions
Xd = [XYd(1); XYd(2)];  % Goal position (same for all AUVs)
XL = [xL; yL];  % Leader positions (one for each AUV)

Rat = norm(Xd - XL);  % Distance to goal

% Initialize output arrays for AUVs
F_psi = zeros(numAUVs, 1);
F_u = zeros(numAUVs, 1);
dist = zeros(numAUVs, 1);

% First repulsion layer (obstacles)
Xobs = [xob(:)'; yob(:)'];
Frep = zeros(2, 4);  % Repulsion force matrix for 4 obstacles

for i = 1:numAUVs
    % For each AUV, calculate the distance to obstacles and apply repulsion
    for j = 1:4
        obs = Xobs(:,j);
        Rrep = norm(obs - XL(:,i)) - R;
        if Rrep <= p0
            F1 = ((1/Rrep) - (1/p0)) * (-(Rat^N)/(Rrep^2));
            F2 = ((1/Rrep) - (1/p0))^2 * (Rat^(N-1));
            Fmag = m*F1 + (N/2)*m*F2;
            dir = atan2(obs(2)-XL(2,i), obs(1)-XL(1,i));
            Frep(:,j) = Fmag * [cos(dir); sin(dir)];
        end
    end
    
    % Calculate total repulsion force for AUV i
    Frep_total = sum(Frep, 2);

    % Calculate attraction force (same goal for all AUVs)
    Fatt = kp * Rat;
    alfa = atan2(Xd(2)-XL(2,i), Xd(1)-XL(1,i));
    Fatt_vec = Fatt * [cos(alfa); sin(alfa)];

    % Total force
    F_total = Frep_total + Fatt_vec;
    F_psi(i) = atan2(F_total(2), F_total(1));  % Heading for AUV i
    F_u(i) = norm(F_total);  % Speed magnitude for AUV i
    dist(i) = norm(Xd - XL(:,i));  % Distance to goal for AUV i
end

end

== matlab function Cooperative/kinematic Moddel1 ==
  data: vr input; psiL input; xdot output; ydot output; u input
function [xdot,ydot] = Position_leader(vr,psiL,u)
% global U0
U0 = u;
% Ucx =0.2; Ucy =0.2; 
Ucx =0.0; Ucy =0.0; 
% Ucx =0.2; Ucy =0.2; 


% x_dot = U0*cos(sa) - vr*sin(sa)+Ucx;
% y_dot = U0*sin(sa) + vr*cos(sa)+Ucy;
xdot  = U0*cos(psiL) - vr*sin(psiL)+ Ucx ;  %x_dot
ydot  = U0*sin(psiL) + vr*cos(psiL)+ Ucy ;  %y_dot

end
